simulink model "servoControl"  (R2024b)
settings: Solver=VariableStepAuto  StartTime=0.0  StopTime=20  RelTol=1e-3
undefined symbols (not defined in the file): A, B, C, K, L, r, t_d, w, x_0
settings Model: Creator=Longbin  LastModifiedBy=Longbin

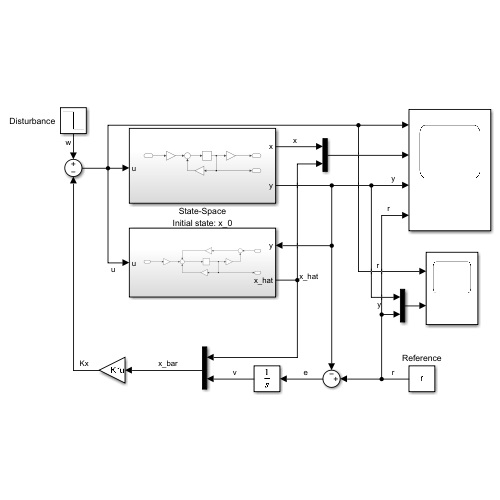
[thumbnail: Simulink's stored preview of the top-level diagram]
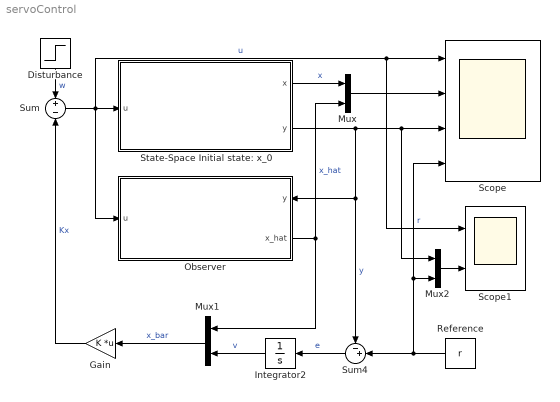
== system servoControl ==
  Disturbance : Step  Time=t_d  After=w  SampleTime=0
  Gain : Gain  Gain=K  Multiplication=Matrix(K*u)
  Integrator2 : Integrator
  Mux : Mux  Inputs=2
  Mux1 : Mux  Inputs=2
  Mux2 : Mux  Inputs=2
  Observer : Subsystem
      settings: PortSchema="{\"entries\":[{\"content\":{\"sides\":[{\"content\":{\"connectorIds\":[\"In1\"]},\"type\":\"ConnectorPlacement.EquallySpacedRectSide\",\"uuid\":\"031d18a1-7477-40ab-8d62-d397f9625b11\"},{\"content\":{\"connectorIds\":[\"In2\",\"Out1\"],\"side\":\"RIGHT\"},\"type\":\"ConnectorPlacement.EquallySpacedRectSide\",\"uuid\":\"2a4462af-6fb1-4aec-a0e4-201ac87307fb\"},{\"content\":{\"side\":\"TOP\"},\"type\":\"ConnectorPlacement.EquallySpacedRectSide\",\"uuid\":\"a47e9843-0fd8-438a-9074-8ef7d54a404a\"}]},\"type\":\"ConnectorPlacement.EquallySpacedConnector\",\"uuid\":\"239d56a6-abdd-4a6f-b55e-120c324b3058\"}],\"packageUris\":[\"http://schema.mathworks.com/mf0/Connector/R2020b\"],\"version\":\"1.0\"}"
  Reference : Constant  Value=r
  Scope : Scope  NumInputPorts=4
  Scope1 : Scope  NumInputPorts=2
  State-Space Initial state: x_0 : Subsystem
  Sum : Sum  Inputs=+|-
  Sum4 : Sum  Inputs=-+|
  wires:
  Gain/1 -> Sum/2  "Kx"
  Sum/1 -> Scope1/1, Scope/1, Observer/1(u), State-Space Initial state: x_0/1(u)  "u"
  Mux/1 -> Scope/2
  Integrator2/1 -> Mux1/2  "v"
  Sum4/1 -> Integrator2/1  "e"
  Reference/1 -> Scope/4, Mux2/2, Sum4/2  "r"
  Mux1/1 -> Gain/1  "x_bar"
  Disturbance/1 -> Sum/1  "w"
  Observer/1(x_hat) -> Mux1/1, Mux/2  "x_hat"
  State-Space Initial state: x_0/2(y) -> Sum4/1, Observer/2(y), Mux2/1, Scope/3  "y"
  State-Space Initial state: x_0/1(x) -> Mux/1  "x"
  Mux2/1 -> Scope1/2

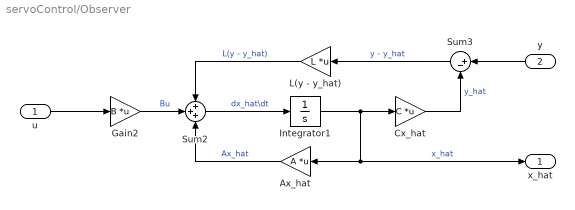
== system servoControl/Observer ==
  u : Inport
  y : Inport  Port=2
  Ax_hat : Gain  Gain=A  Multiplication=Matrix(K*u)
  Cx_hat : Gain  Gain=C  Multiplication=Matrix(K*u)
  Gain2 : Gain  Gain=B  Multiplication=Matrix(K*u)
  Integrator1 : Integrator
  L(y - y_hat) : Gain  Gain=L  Multiplication=Matrix(K*u)
  Sum2 : Sum  Inputs=+++
  Sum3 : Sum  Inputs=|+-
  x_hat : Outport
  wires:
  Cx_hat/1 -> Sum3/2  "y_hat"
  Gain2/1 -> Sum2/2  "Bu"
  L(y - y_hat)/1 -> Sum2/1  "L(y - y_hat)"
  Sum2/1 -> Integrator1/1  "dx_hat\\dt"
  Ax_hat/1 -> Sum2/3  "Ax_hat"
  Integrator1/1 -> Ax_hat/1, x_hat/1, Cx_hat/1  "x_hat"
  Sum3/1 -> L(y - y_hat)/1  "y - y_hat"
  y/1 -> Sum3/1
  u/1 -> Gain2/1

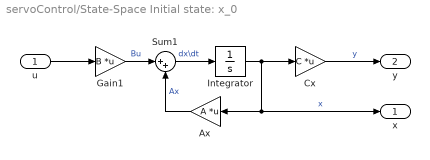
== system servoControl/State-Space Initial state: x_0 ==
  u : Inport
  Ax : Gain  Gain=A  Multiplication=Matrix(K*u)
  Cx : Gain  Gain=C  Multiplication=Matrix(K*u)
  Gain1 : Gain  Gain=B  Multiplication=Matrix(K*u)
  Integrator : Integrator  InitialCondition=x_0
  Sum1 : Sum  Inputs=|++
  x : Outport
  y : Outport  Port=2
  wires:
  Gain1/1 -> Sum1/1  "Bu"
  u/1 -> Gain1/1
  Ax/1 -> Sum1/2  "Ax"
  Sum1/1 -> Integrator/1  "dx\\dt"
  Integrator/1 -> Cx/1, x/1, Ax/1  "x"
  Cx/1 -> y/1  "y"
